simulink model "unipolar_spwm_inverter"  (R2022a)
settings: Solver=ode23tb  StartTime=0.0  StopTime=0.04  RelTol=1e-3
libraries: spsIGBTDiodeLib x4, spsTriangleGeneratorLib x2, spsDCVoltageSourceLib x1, spsSeriesRLCBranchLib x1, spsVoltageMeasurementLib x1, spspowerguiLib x1
settings Model: Creator=asher  LastModifiedBy=asher
settings DataIOCC: ReturnWorkspaceOutputs=off

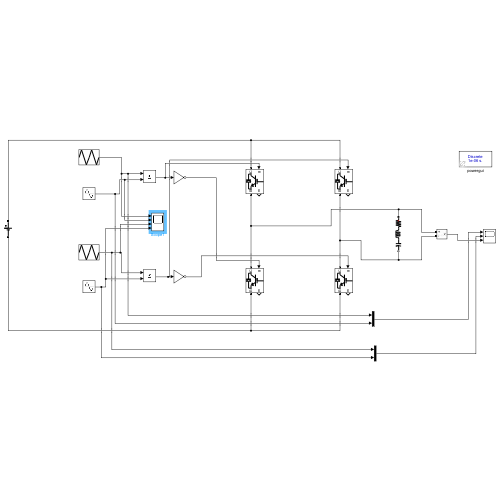
[thumbnail: Simulink's stored preview of the top-level diagram]
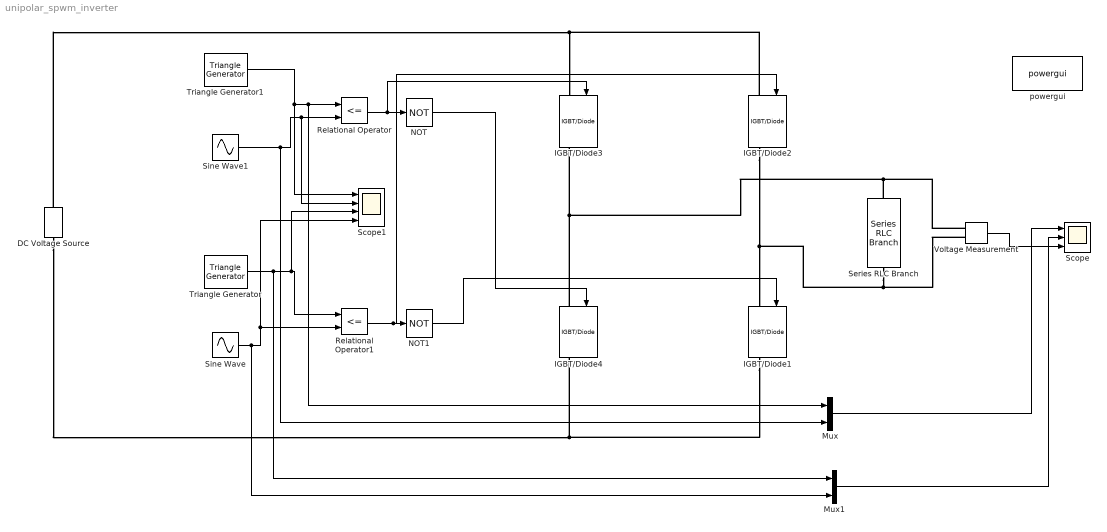
== system unipolar_spwm_inverter ==
  DC Voltage Source : spsDCVoltageSourceLib/DC Voltage Source  Amplitude=300  Measurements=None
  IGBT/Diode{1..4} (4 alike) : spsIGBTDiodeLib/IGBT//Diode  Ron=1e-3  Rs=1e5  Cs=inf  Measurements=on
  Mux : Mux  Inputs=2
  Mux1 : Mux  Inputs=2
  NOT : Logic  Operator=NOT  IconShape=distinctive  AllPortsSameDT=off  OutDataTypeStr=boolean
  NOT1 : Logic  Operator=NOT  IconShape=distinctive  AllPortsSameDT=off  OutDataTypeStr=boolean
  Relational Operator : RelationalOperator  Operator=<=  OutDataTypeStr=boolean  RndMeth=Simplest  InputSameDT=off
  Relational Operator1 : RelationalOperator  Operator=<=  OutDataTypeStr=boolean  RndMeth=Simplest  InputSameDT=off
  Scope : Scope  NumInputPorts=3
  Scope1 : Scope  NumInputPorts=4
  Series RLC Branch : spsSeriesRLCBranchLib/Series RLC Branch  LConnTagsString=__new0  RConnTagsString=__new0  BranchType=RLC  Resistance=1  Inductance=1e-3  SetiL0=off  InitialCurrent=0  Capacitance=1e-6  Setx0=off  InitialVoltage=0  Measurements=None
  Sine Wave : Sin  Amplitude=0.9  Frequency=2*pi*50  Phase=pi  SampleTime=0
  Sine Wave1 : Sin  Amplitude=0.9  Frequency=2*pi*50  SampleTime=0
  Triangle Generator : spsTriangleGeneratorLib/Triangle Generator  Freq=1e3  Phase=90  Ts=0
  Triangle Generator1 : spsTriangleGeneratorLib/Triangle Generator  Freq=1e3  Phase=90  Ts=0
  Voltage Measurement : spsVoltageMeasurementLib/Voltage Measurement  PhasorSimulation=off  OutputType=Complex  PSBequivalent=0
  powergui : spspowerguiLib/powergui  Priority=1  SimulationMode=Discrete  SampleTime=1e-6  frequency=60  Iterations=50  frequencyindice=0  Pbase=100e6  ErrMax=1e-4  UnitsV=kV  UnitsW=MW  buscounter=0  FunctionMessages=off  echomessages=off  EnableUseOfTLC=off  CurrentSourceSwitches=off  DisableSnubberDevices=off  DisableRonSwitches=off  DisableVfSwitches=off  DisplayEquations=off  AutomaticDiscreteSolvers=off  SolverType=Tustin/Backward Euler (TBE)  Interpol=off  ExternalGateDelay=off  methode=off  Ts=100  x0status=blocks  SPID=on  SwTol=0  HookPort=off  NonlinearTolerance=1e-4  nMaxIteration=100  ContinueOnMaxIteration=off  RestoreLinks=warning  ResistiveCurrentMeasurement=off  Frange=[0:2:500]  Ylog=off  Xlog=on  ShowGrid=off  save=off  variable=ZData  structure=0  ZoomFFT=off  StartTime=0.0  cycles=1  DisplayStyle=1  fundamental=60  FreqAxis=off  MaxFrequency=1000  frequencyindicesteady=1  RmsSteady=1  display=off
  wires:
  Voltage Measurement/1 -> Scope/3
  Sine Wave1/1 -> Mux/2, Scope1/2, Relational Operator/2
  Triangle Generator1/1 -> Scope1/1, Mux/1, Relational Operator/1
  Relational Operator/1 -> IGBT/Diode3/1, NOT/1
  Triangle Generator/1 -> Mux1/1, Scope1/3, Relational Operator1/1
  Relational Operator1/1 -> IGBT/Diode2/1, NOT1/1
  NOT/1 -> IGBT/Diode4/1
  NOT1/1 -> IGBT/Diode1/1
  Mux1/1 -> Scope/2
  Mux/1 -> Scope/1
  Sine Wave/1 -> Mux1/2, Relational Operator1/2, Scope1/4
  connections:
  DC Voltage Source/RConn1 -- IGBT/Diode2/LConn1 -- IGBT/Diode3/LConn1
  DC Voltage Source/LConn1 -- IGBT/Diode1/RConn1 -- IGBT/Diode4/RConn1
  IGBT/Diode4/LConn1 -- Voltage Measurement/LConn1 -- Series RLC Branch/LConn1 -- IGBT/Diode3/RConn1
  IGBT/Diode2/RConn1 -- Voltage Measurement/LConn2 -- Series RLC Branch/RConn1 -- IGBT/Diode1/LConn1
